simulink model "calcul_SA_SR"  (R2024b)
settings: Solver=FixedStepAuto  StartTime=0.0  StopTime=10.0  FixedStep=Ts  RelTol=1e-3
values from neighbouring files (symbols this model uses):
  Re = 0.47/2    (= 0.235)    [main_data_vehicle.m]
settings Model: Creator=marti  LastModifiedBy=marti

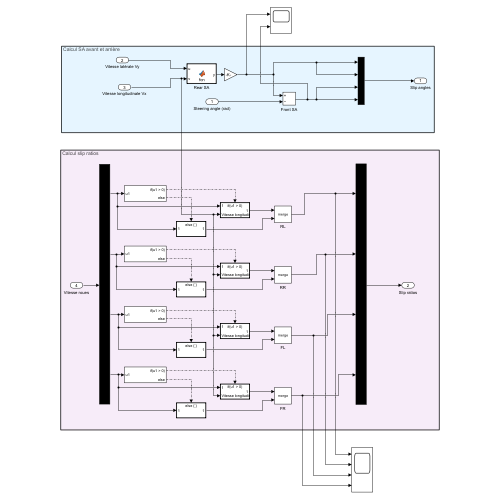
[thumbnail: Simulink's stored preview of the top-level diagram]
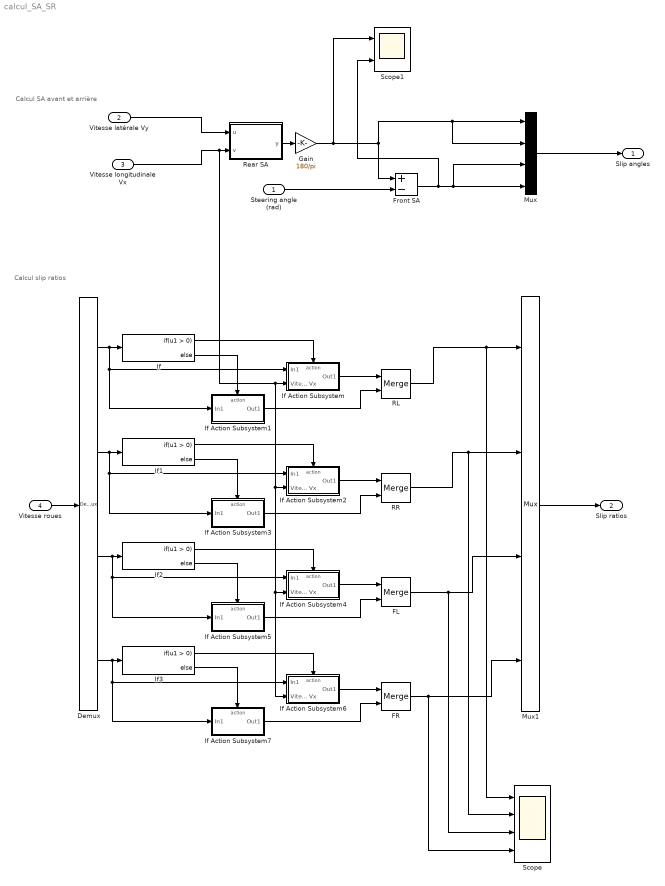
== system calcul_SA_SR ==
  note: Calcul SA avant et arrière
  note: Calcul slip ratios
  Steering angle (rad) : Inport
  Vitesse latérale Vy : Inport  Port=2
  Vitesse longitudinale Vx : Inport  Port=3
  Vitesse roues : Inport  Port=4
  Demux : Demux
  FL : Merge
  FR : Merge
  Front SA : Sum  Inputs=+-
  Gain : Gain  Gain=180/pi
  If{,1..3} (4 alike) : If
  If Action Subsystem : Subsystem  TreatAsAtomicUnit=on
  If Action Subsystem1 : Subsystem  TreatAsAtomicUnit=on
  If Action Subsystem2 : Subsystem  TreatAsAtomicUnit=on
  If Action Subsystem3 : Subsystem  TreatAsAtomicUnit=on
  If Action Subsystem4 : Subsystem  TreatAsAtomicUnit=on
  If Action Subsystem5 : Subsystem  TreatAsAtomicUnit=on
  If Action Subsystem6 : Subsystem  TreatAsAtomicUnit=on
  If Action Subsystem7 : Subsystem  TreatAsAtomicUnit=on
  Mux : Mux
  Mux1 : Mux
  RL : Merge
  RR : Merge
  Rear SA : MATLAB Function  TreatAsAtomicUnit=on
  Scope : Scope  NumInputPorts=4
  Scope1 : Scope  NumInputPorts=2
  Slip angles : Outport
  Slip ratios : Outport  Port=2
  wires:
  Vitesse latérale Vy/1 -> Rear SA/1(u)
  Steering angle (rad)/1 -> Front SA/2
  Rear SA/1(y) -> Gain/1
  Front SA/1 -> Scope1/2, Mux/3, Mux/4
  Mux/1 -> Slip angles/1
  Mux1/1 -> Slip ratios/1
  Vitesse roues/1 -> Demux/1
  Vitesse longitudinale Vx/1 -> If Action Subsystem6/2(Vitesse longitudinale Vx), If Action Subsystem4/2(Vitesse longitudinale Vx), If Action Subsystem2/2(Vitesse longitudinale Vx), If Action Subsystem/2(Vitesse longitudinale Vx), Rear SA/2(v)
  Demux/1 -> If Action Subsystem1/1(In1), If Action Subsystem/1(In1), If/1
  If/1 -> If Action Subsystem/Action
  If/2 -> If Action Subsystem1/Action
  If Action Subsystem/1(Out1) -> RL/1
  If Action Subsystem1/1(Out1) -> RL/2
  If1/1 -> If Action Subsystem2/Action
  If Action Subsystem2/1(Out1) -> RR/1
  If Action Subsystem3/1(Out1) -> RR/2
  Demux/2 -> If Action Subsystem3/1(In1), If Action Subsystem2/1(In1), If1/1
  If1/2 -> If Action Subsystem3/Action
  If2/1 -> If Action Subsystem4/Action
  If Action Subsystem4/1(Out1) -> FL/1
  If Action Subsystem5/1(Out1) -> FL/2
  Demux/3 -> If Action Subsystem5/1(In1), If Action Subsystem4/1(In1), If2/1
  If2/2 -> If Action Subsystem5/Action
  If3/1 -> If Action Subsystem6/Action
  If Action Subsystem6/1(Out1) -> FR/1
  If Action Subsystem7/1(Out1) -> FR/2
  Demux/4 -> If Action Subsystem7/1(In1), If Action Subsystem6/1(In1), If3/1
  If3/2 -> If Action Subsystem7/Action
  RL/1 -> Scope/1, Mux1/1
  RR/1 -> Scope/2, Mux1/2
  FL/1 -> Scope/3, Mux1/3
  FR/1 -> Scope/4, Mux1/4
  Gain/1 -> Scope1/1, Front SA/1, Mux/2, Mux/1

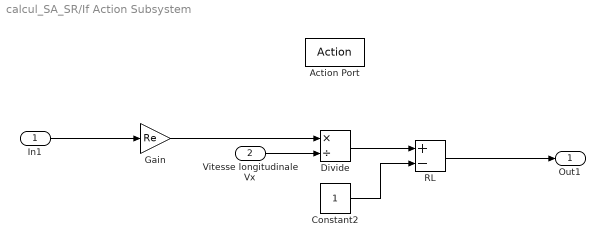
== system calcul_SA_SR/If Action Subsystem ==
  In1 : Inport
  Vitesse longitudinale Vx : Inport  Port=2
  Action Port : ActionPort  ActionPortLabel=if(u1 > 0)
  Constant2 : Constant
  Divide : Product  Inputs=*/
  Gain : Gain  Gain=Re
  RL : Sum  Inputs=+-
  Out1 : Outport
  wires:
  Vitesse longitudinale Vx/1 -> Divide/2
  Divide/1 -> RL/1
  RL/1 -> Out1/1
  Constant2/1 -> RL/2
  In1/1 -> Gain/1
  Gain/1 -> Divide/1

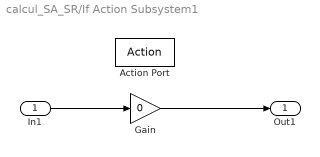
== system calcul_SA_SR/If Action Subsystem1 ==
  In1 : Inport
  Action Port : ActionPort  ActionPortLabel=else
  Gain : Gain  Gain=0
  Out1 : Outport
  wires:
  In1/1 -> Gain/1
  Gain/1 -> Out1/1

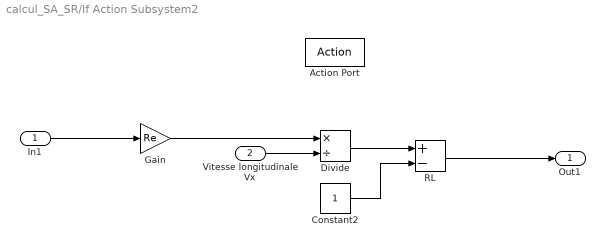
== system calcul_SA_SR/If Action Subsystem2 ==
  In1 : Inport
  Vitesse longitudinale Vx : Inport  Port=2
  Action Port : ActionPort  ActionPortLabel=if(u1 > 0)
  Constant2 : Constant
  Divide : Product  Inputs=*/
  Gain : Gain  Gain=Re
  RL : Sum  Inputs=+-
  Out1 : Outport
  wires:
  Vitesse longitudinale Vx/1 -> Divide/2
  Divide/1 -> RL/1
  RL/1 -> Out1/1
  Constant2/1 -> RL/2
  In1/1 -> Gain/1
  Gain/1 -> Divide/1

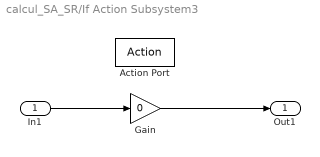
== system calcul_SA_SR/If Action Subsystem3 ==
  In1 : Inport
  Action Port : ActionPort  ActionPortLabel=else
  Gain : Gain  Gain=0
  Out1 : Outport
  wires:
  In1/1 -> Gain/1
  Gain/1 -> Out1/1

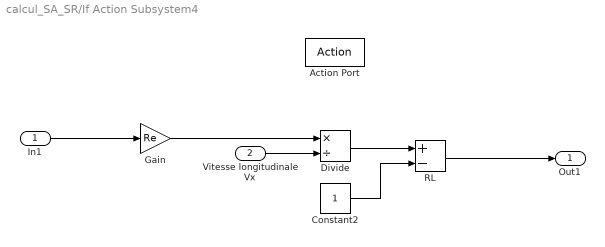
== system calcul_SA_SR/If Action Subsystem4 ==
  In1 : Inport
  Vitesse longitudinale Vx : Inport  Port=2
  Action Port : ActionPort  ActionPortLabel=if(u1 > 0)
  Constant2 : Constant
  Divide : Product  Inputs=*/
  Gain : Gain  Gain=Re
  RL : Sum  Inputs=+-
  Out1 : Outport
  wires:
  Vitesse longitudinale Vx/1 -> Divide/2
  Divide/1 -> RL/1
  RL/1 -> Out1/1
  Constant2/1 -> RL/2
  In1/1 -> Gain/1
  Gain/1 -> Divide/1

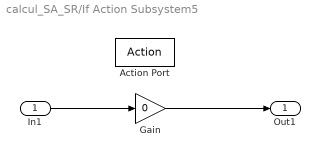
== system calcul_SA_SR/If Action Subsystem5 ==
  In1 : Inport
  Action Port : ActionPort  ActionPortLabel=else
  Gain : Gain  Gain=0
  Out1 : Outport
  wires:
  In1/1 -> Gain/1
  Gain/1 -> Out1/1

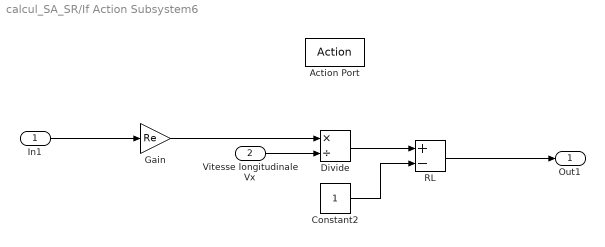
== system calcul_SA_SR/If Action Subsystem6 ==
  In1 : Inport
  Vitesse longitudinale Vx : Inport  Port=2
  Action Port : ActionPort  ActionPortLabel=if(u1 > 0)
  Constant2 : Constant
  Divide : Product  Inputs=*/
  Gain : Gain  Gain=Re
  RL : Sum  Inputs=+-
  Out1 : Outport
  wires:
  Vitesse longitudinale Vx/1 -> Divide/2
  Divide/1 -> RL/1
  RL/1 -> Out1/1
  Constant2/1 -> RL/2
  In1/1 -> Gain/1
  Gain/1 -> Divide/1

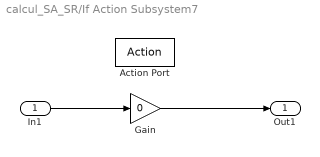
== system calcul_SA_SR/If Action Subsystem7 ==
  In1 : Inport
  Action Port : ActionPort  ActionPortLabel=else
  Gain : Gain  Gain=0
  Out1 : Outport
  wires:
  In1/1 -> Gain/1
  Gain/1 -> Out1/1

== matlab function calcul_SA_SR/Rear SA ==
  data: u input; y output; v input
function y = fcn(u, v)

y = atan(u/v);
end
